simulink model "EMS"  (R2024b)
settings: configuration reference "STM32H7_Config" (kept outside this file)
undefined symbols (not defined in the file): rEMSTarget
libraries: simulink x4
settings Model: DataDictionary=Master_Dictionary.sldd  EnableAccessToBaseWorkspace=off  Creator=torni  LastModifiedBy=William
settings ConfigSetRef: SourceName=STM32H7_Config

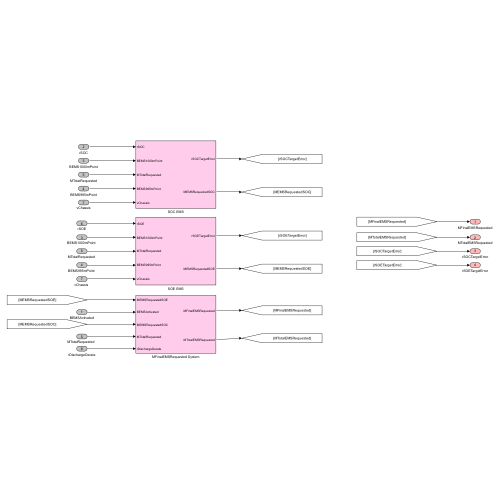
[thumbnail: Simulink's stored preview of the top-level diagram]
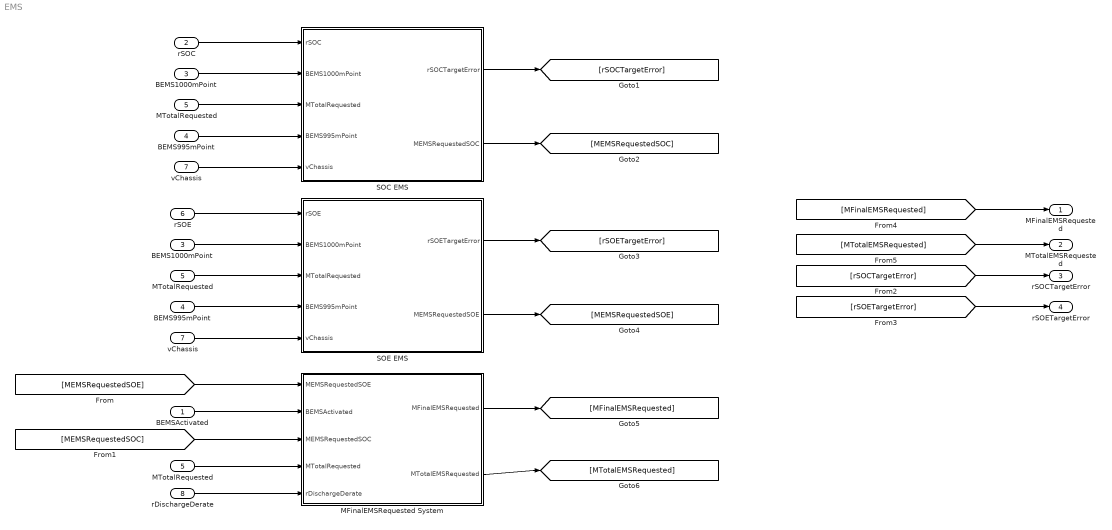
== system EMS ==
  BEMSActivated : Inport  OutDataTypeStr=boolean
  rSOC : Inport  Port=2  OutDataTypeStr=double
  BEMS1000mPoint : Inport  Port=3  OutDataTypeStr=boolean
  BEMS995mPoint : Inport  Port=4  OutDataTypeStr=boolean
  MTotalRequested : Inport  Port=5  OutDataTypeStr=double
  rSOE : Inport  Port=6  OutDataTypeStr=double
  vChassis : Inport  Port=7  OutDataTypeStr=double
  rDischargeDerate : Inport  Port=8  OutDataTypeStr=double
  "BEMS1000mPoint " : InportShadow  Port=3  OutDataTypeStr=boolean
  "BEMS995mPoint " : InportShadow  Port=4  OutDataTypeStr=boolean
  MFinalEMSRequested System : Subsystem
  "MTotalRequested " : InportShadow  Port=5  OutDataTypeStr=double
  "MTotalRequested  " : InportShadow  Port=5  OutDataTypeStr=double
  SOC EMS : Subsystem
  SOE EMS : Subsystem
  "vChassis " : InportShadow  Port=7  OutDataTypeStr=double
  MFinalEMSRequested : Outport  OutDataTypeStr=double  VectorParamsAs1DForOutWhenUnconnected=off
  MTotalEMSRequested : Outport  Port=2  OutDataTypeStr=double  VectorParamsAs1DForOutWhenUnconnected=off
  rSOCTargetError : Outport  Port=3  OutDataTypeStr=double  VectorParamsAs1DForOutWhenUnconnected=off
  rSOETargetError : Outport  Port=4  OutDataTypeStr=double  VectorParamsAs1DForOutWhenUnconnected=off
  wires:
  [rSOETargetError] -> rSOETargetError/1
  [rSOCTargetError] -> rSOCTargetError/1
  rSOC/1 -> SOC EMS/1(rSOC)
  BEMS1000mPoint/1 -> SOC EMS/2(BEMS1000mPoint)
  BEMS995mPoint/1 -> SOC EMS/4(BEMS995mPoint)
  MTotalRequested/1 -> SOC EMS/3(MTotalRequested)
  rSOE/1 -> SOE EMS/1(rSOE)
  "BEMS1000mPoint "/1 -> SOE EMS/2(BEMS1000mPoint)
  "BEMS995mPoint "/1 -> SOE EMS/4(BEMS995mPoint)
  "MTotalRequested "/1 -> SOE EMS/3(MTotalRequested)
  SOC EMS/1(rSOCTargetError) -> [rSOCTargetError]
  SOC EMS/2(MEMSRequestedSOC) -> [MEMSRequestedSOC]
  SOE EMS/1(rSOETargetError) -> [rSOETargetError]
  SOE EMS/2(MEMSRequestedSOE) -> [MEMSRequestedSOE]
  BEMSActivated/1 -> MFinalEMSRequested System/2(BEMSActivated)
  "MTotalRequested  "/1 -> MFinalEMSRequested System/4(MTotalRequested)
  [MEMSRequestedSOE] -> MFinalEMSRequested System/1(MEMSRequestedSOE)
  [MEMSRequestedSOC] -> MFinalEMSRequested System/3(MEMSRequestedSOC)
  MFinalEMSRequested System/1(MFinalEMSRequested) -> [MFinalEMSRequested]
  MFinalEMSRequested System/2(MTotalEMSRequested) -> [MTotalEMSRequested]
  [MFinalEMSRequested] -> MFinalEMSRequested/1
  [MTotalEMSRequested] -> MTotalEMSRequested/1
  vChassis/1 -> SOC EMS/5(vChassis)
  "vChassis "/1 -> SOE EMS/5(vChassis)
  rDischargeDerate/1 -> MFinalEMSRequested System/5(rDischargeDerate)

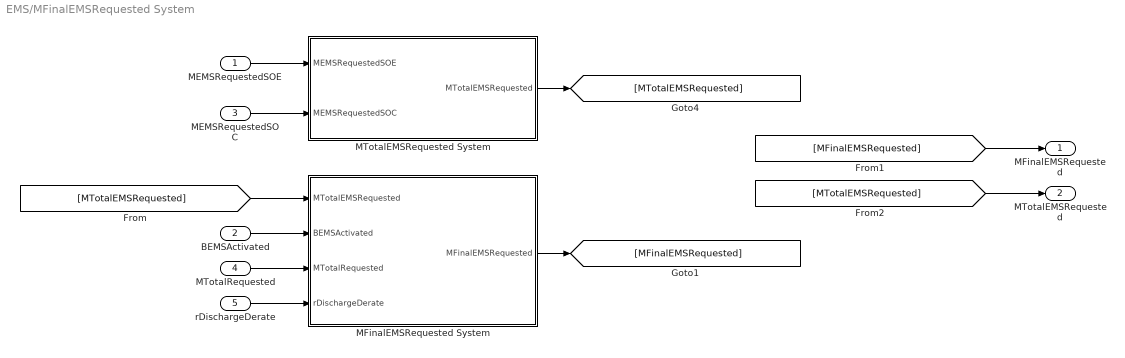
== system EMS/MFinalEMSRequested System ==
  MEMSRequestedSOE : Inport  OutDataTypeStr=double
  BEMSActivated : Inport  Port=2  OutDataTypeStr=boolean
  MEMSRequestedSOC : Inport  Port=3  OutDataTypeStr=double
  MTotalRequested : Inport  Port=4  OutDataTypeStr=double
  rDischargeDerate : Inport  Port=5  OutDataTypeStr=double
  MFinalEMSRequested System : Subsystem
  MTotalEMSRequested System : Subsystem
  MFinalEMSRequested : Outport  OutDataTypeStr=double  VectorParamsAs1DForOutWhenUnconnected=off
  MTotalEMSRequested : Outport  Port=2  OutDataTypeStr=double  VectorParamsAs1DForOutWhenUnconnected=off
  wires:
  [MTotalEMSRequested] -> MTotalEMSRequested/1
  MEMSRequestedSOE/1 -> MTotalEMSRequested System/1(MEMSRequestedSOE)
  MEMSRequestedSOC/1 -> MTotalEMSRequested System/2(MEMSRequestedSOC)
  MTotalEMSRequested System/1(MTotalEMSRequested) -> [MTotalEMSRequested]
  BEMSActivated/1 -> MFinalEMSRequested System/2(BEMSActivated)
  MTotalRequested/1 -> MFinalEMSRequested System/3(MTotalRequested)
  MFinalEMSRequested System/1(MFinalEMSRequested) -> [MFinalEMSRequested]
  [MTotalEMSRequested] -> MFinalEMSRequested System/1(MTotalEMSRequested)
  [MFinalEMSRequested] -> MFinalEMSRequested/1
  rDischargeDerate/1 -> MFinalEMSRequested System/4(rDischargeDerate)

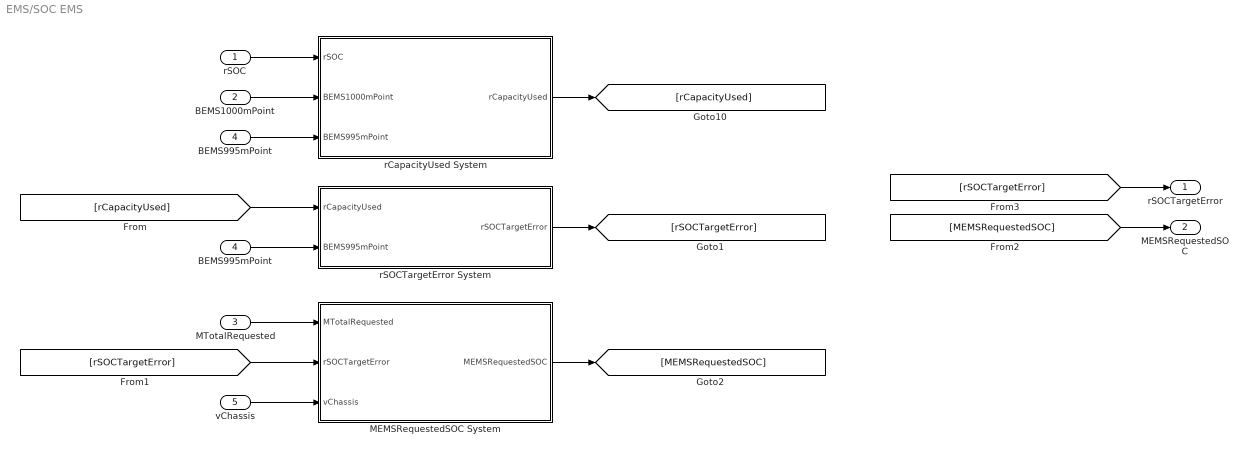
== system EMS/SOC EMS ==
  rSOC : Inport  OutDataTypeStr=double
  BEMS1000mPoint : Inport  Port=2  OutDataTypeStr=boolean
  MTotalRequested : Inport  Port=3  OutDataTypeStr=double
  BEMS995mPoint : Inport  Port=4  OutDataTypeStr=boolean
  vChassis : Inport  Port=5  OutDataTypeStr=double
  "BEMS995mPoint " : InportShadow  Port=4  OutDataTypeStr=boolean
  MEMSRequestedSOC System : Subsystem
  rCapacityUsed System : Subsystem
  rSOCTargetError System : Subsystem
  rSOCTargetError : Outport  OutDataTypeStr=double  VectorParamsAs1DForOutWhenUnconnected=off
  MEMSRequestedSOC : Outport  Port=2  OutDataTypeStr=double
  wires:
  BEMS995mPoint/1 -> rCapacityUsed System/3(BEMS995mPoint)
  MTotalRequested/1 -> MEMSRequestedSOC System/1(MTotalRequested)
  MEMSRequestedSOC System/1(MEMSRequestedSOC) -> [MEMSRequestedSOC]
  BEMS1000mPoint/1 -> rCapacityUsed System/2(BEMS1000mPoint)
  rSOC/1 -> rCapacityUsed System/1(rSOC)
  rCapacityUsed System/1(rCapacityUsed) -> [rCapacityUsed]
  [rCapacityUsed] -> rSOCTargetError System/1(rCapacityUsed)
  "BEMS995mPoint "/1 -> rSOCTargetError System/2(BEMS995mPoint)
  rSOCTargetError System/1(rSOCTargetError) -> [rSOCTargetError]
  [rSOCTargetError] -> MEMSRequestedSOC System/2(rSOCTargetError)
  [MEMSRequestedSOC] -> MEMSRequestedSOC/1
  [rSOCTargetError] -> rSOCTargetError/1
  vChassis/1 -> MEMSRequestedSOC System/3(vChassis)

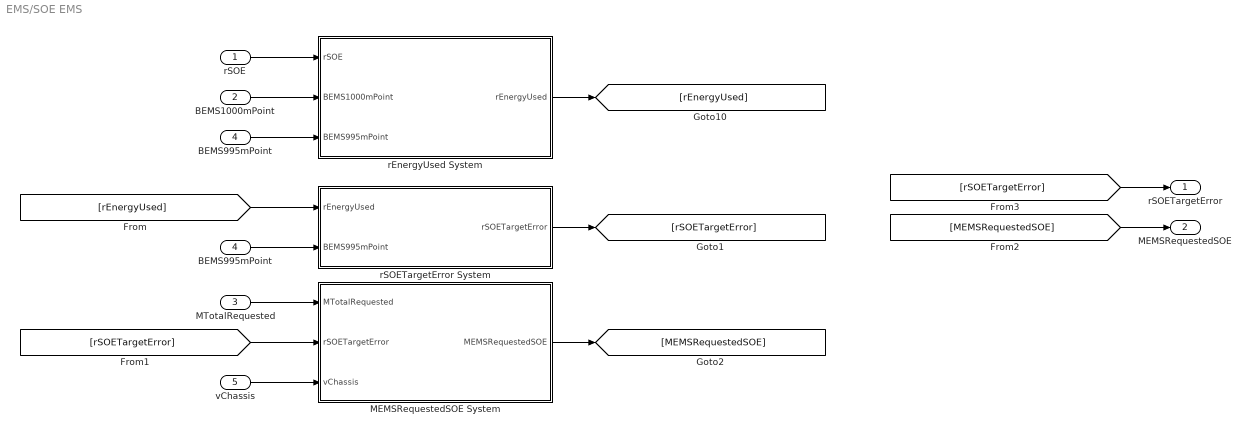
== system EMS/SOE EMS ==
  rSOE : Inport  OutDataTypeStr=double
  BEMS1000mPoint : Inport  Port=2  OutDataTypeStr=boolean
  MTotalRequested : Inport  Port=3  OutDataTypeStr=double
  BEMS995mPoint : Inport  Port=4  OutDataTypeStr=boolean
  vChassis : Inport  Port=5  OutDataTypeStr=double
  "BEMS995mPoint " : InportShadow  Port=4  OutDataTypeStr=boolean
  MEMSRequestedSOE System : Subsystem
  rEnergyUsed System : Subsystem
  rSOETargetError System : Subsystem
  rSOETargetError : Outport  OutDataTypeStr=double  VectorParamsAs1DForOutWhenUnconnected=off
  MEMSRequestedSOE : Outport  Port=2  OutDataTypeStr=double
  wires:
  [rSOETargetError] -> rSOETargetError/1
  [MEMSRequestedSOE] -> MEMSRequestedSOE/1
  [rSOETargetError] -> MEMSRequestedSOE System/2(rSOETargetError)
  rSOETargetError System/1(rSOETargetError) -> [rSOETargetError]
  "BEMS995mPoint "/1 -> rSOETargetError System/2(BEMS995mPoint)
  [rEnergyUsed] -> rSOETargetError System/1(rEnergyUsed)
  rEnergyUsed System/1(rEnergyUsed) -> [rEnergyUsed]
  rSOE/1 -> rEnergyUsed System/1(rSOE)
  BEMS1000mPoint/1 -> rEnergyUsed System/2(BEMS1000mPoint)
  MEMSRequestedSOE System/1(MEMSRequestedSOE) -> [MEMSRequestedSOE]
  MTotalRequested/1 -> MEMSRequestedSOE System/1(MTotalRequested)
  BEMS995mPoint/1 -> rEnergyUsed System/3(BEMS995mPoint)
  vChassis/1 -> MEMSRequestedSOE System/3(vChassis)

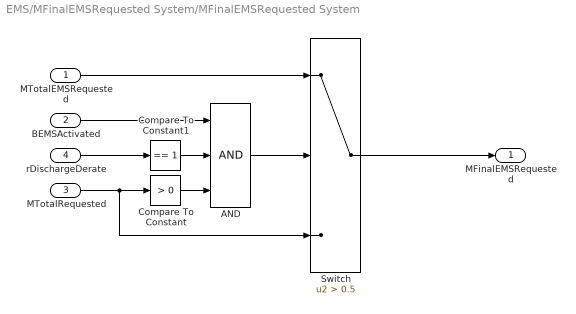
== system EMS/MFinalEMSRequested System/MFinalEMSRequested System ==
  MTotalEMSRequested : Inport  OutDataTypeStr=double
  BEMSActivated : Inport  Port=2  OutDataTypeStr=boolean
  MTotalRequested : Inport  Port=3  OutDataTypeStr=double
  rDischargeDerate : Inport  Port=4  OutDataTypeStr=double
  AND : Logic  Inputs=3  AllPortsSameDT=off  OutDataTypeStr=boolean
  Compare To Constant : simulink/Logic and Bit Operations/Compare To Constant  relop=>  const=0  OutDataTypeStr=boolean
  Compare To Constant1 : simulink/Logic and Bit Operations/Compare To Constant  relop===  const=1  OutDataTypeStr=boolean
  Switch : Switch  Criteria=u2 > Threshold  Threshold=0.5  SaturateOnIntegerOverflow=off  InputSameDT=off
  MFinalEMSRequested : Outport  OutDataTypeStr=double  VectorParamsAs1DForOutWhenUnconnected=off
  wires:
  MTotalEMSRequested/1 -> Switch/1
  MTotalRequested/1 -> Switch/3, Compare To Constant/1
  AND/1 -> Switch/2
  BEMSActivated/1 -> AND/1
  Switch/1 -> MFinalEMSRequested/1
  Compare To Constant/1 -> AND/3
  rDischargeDerate/1 -> Compare To Constant1/1
  Compare To Constant1/1 -> AND/2

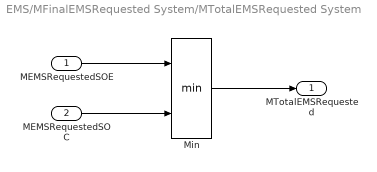
== system EMS/MFinalEMSRequested System/MTotalEMSRequested System ==
  MEMSRequestedSOE : Inport  OutDataTypeStr=double
  MEMSRequestedSOC : Inport  Port=2  OutDataTypeStr=double
  Min : MinMax  Inputs=2
  MTotalEMSRequested : Outport  OutDataTypeStr=double  VectorParamsAs1DForOutWhenUnconnected=off
  wires:
  MEMSRequestedSOE/1 -> Min/1
  MEMSRequestedSOC/1 -> Min/2
  Min/1 -> MTotalEMSRequested/1

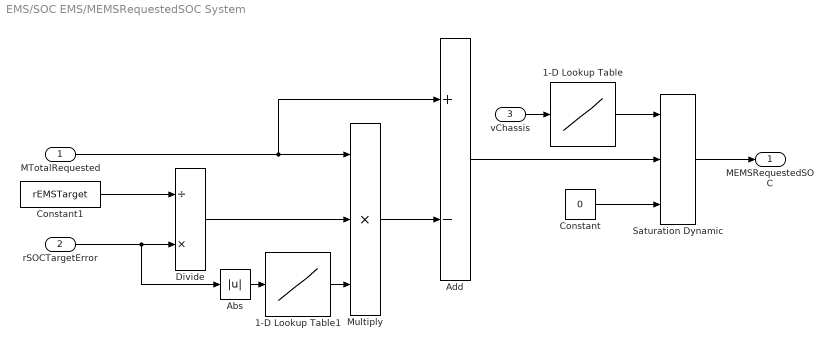
== system EMS/SOC EMS/MEMSRequestedSOC System ==
  MTotalRequested : Inport  OutDataTypeStr=double
  rSOCTargetError : Inport  Port=2  OutDataTypeStr=double
  vChassis : Inport  Port=3  OutDataTypeStr=double
  1-D Lookup Table : Lookup_n-D  NumberOfTableDimensions=1  BreakpointsForDimension1=|  Table=|  InternalRulePriority=Speed  RndMeth=Simplest
      BreakpointsForDimension1=|
      | [0.00
      | 1.37
      | 2.73
      | 4.10
      | 5.47
      | 6.84
      | 8.20
      | 9.57
      | 10.94
      | 12.30
      | 13.67
      | 15.04
      | 16.40
      | 17.77
      | 19.14
      | 20.51
      | 21.87
      | 23.24
      | 24.61
      | 25.97
      | 27.34]
      Table=|
      | [583.09
      | 583.09
      | 583.09
      | 583.09
      | 583.09
      | 583.09
      | 583.09
      | 583.09
      | 583.09
      | 583.09
      | 583.09
      | 523.483965
      | 463.877551
      | 463.877551
      | 463.877551
      | 463.877551
      | 463.877551
      | 463.877551
      | 463.877551
      | 463.877551
      | 463.877551]
  1-D Lookup Table1 : Lookup_n-D  NumberOfTableDimensions=1  BreakpointsForDimension1=[0 5]  Table=[0 3.8]  InternalRulePriority=Speed  RndMeth=Simplest
  Abs : Abs  SaturateOnIntegerOverflow=off
  Add : Sum  Inputs=+-
  Constant : Constant  Value=0
  Constant1 : Constant  Value=rEMSTarget
  Divide : Product  Inputs=/*
  Multiply : Product  Inputs=3
  Saturation Dynamic : simulink/Discontinuities/Saturation Dynamic  OutMin=[]  OutMax=[]  OutDataTypeStr=Inherit: Same as second input  OutDataType=fixdt(1, 16)  OutScaling=2^-10  DoSatur=off
  MEMSRequestedSOC : Outport  OutDataTypeStr=double
  wires:
  MTotalRequested/1 -> Add/1, Multiply/1
  Divide/1 -> Multiply/2
  Constant1/1 -> Divide/1
  rSOCTargetError/1 -> Abs/1, Divide/2
  Multiply/1 -> Add/2
  Add/1 -> Saturation Dynamic/2
  Saturation Dynamic/1 -> MEMSRequestedSOC/1
  1-D Lookup Table1/1 -> Multiply/3
  1-D Lookup Table/1 -> Saturation Dynamic/1
  vChassis/1 -> 1-D Lookup Table/1
  Constant/1 -> Saturation Dynamic/3
  Abs/1 -> 1-D Lookup Table1/1

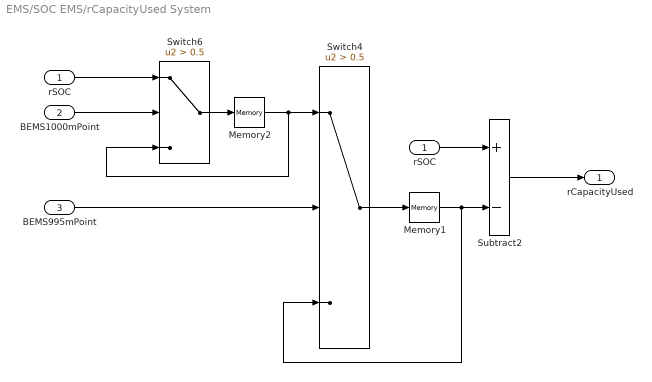
== system EMS/SOC EMS/rCapacityUsed System ==
  rSOC : Inport  OutDataTypeStr=double
  BEMS1000mPoint : Inport  Port=2  OutDataTypeStr=boolean
  BEMS995mPoint : Inport  Port=3  OutDataTypeStr=boolean
  Memory1 : Memory  InitialCondition=100  InheritSampleTime=on
  Memory2 : Memory  InitialCondition=100  InheritSampleTime=on
  Subtract2 : Sum  Inputs=+-
  Switch4 : Switch  Criteria=u2 > Threshold  Threshold=0.5  SaturateOnIntegerOverflow=off  InputSameDT=off
  Switch6 : Switch  Criteria=u2 > Threshold  Threshold=0.5  SaturateOnIntegerOverflow=off  InputSameDT=off
  "rSOC " : InportShadow  OutDataTypeStr=double
  rCapacityUsed : Outport  OutDataTypeStr=double  VectorParamsAs1DForOutWhenUnconnected=off
  wires:
  BEMS1000mPoint/1 -> Switch6/2
  Memory1/1 -> Switch4/3, Subtract2/2
  Switch4/1 -> Memory1/1
  BEMS995mPoint/1 -> Switch4/2
  rSOC/1 -> Switch6/1
  Switch6/1 -> Memory2/1
  Subtract2/1 -> rCapacityUsed/1
  Memory2/1 -> Switch6/3, Switch4/1
  "rSOC "/1 -> Subtract2/1

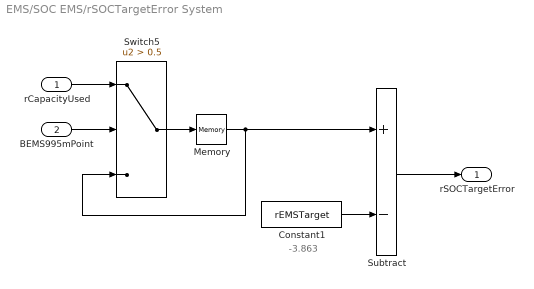
== system EMS/SOC EMS/rSOCTargetError System ==
  note: -3.863
  rCapacityUsed : Inport  OutDataTypeStr=double
  BEMS995mPoint : Inport  Port=2  OutDataTypeStr=boolean
  Constant1 : Constant  Value=rEMSTarget
  Memory : Memory  InitialCondition=-3.863  InheritSampleTime=on
  Subtract : Sum  Inputs=+-
  Switch5 : Switch  Criteria=u2 > Threshold  Threshold=0.5  SaturateOnIntegerOverflow=off  InputSameDT=off
  rSOCTargetError : Outport  OutDataTypeStr=double  VectorParamsAs1DForOutWhenUnconnected=off
  wires:
  rCapacityUsed/1 -> Switch5/1
  Switch5/1 -> Memory/1
  Constant1/1 -> Subtract/2
  BEMS995mPoint/1 -> Switch5/2
  Memory/1 -> Switch5/3, Subtract/1
  Subtract/1 -> rSOCTargetError/1

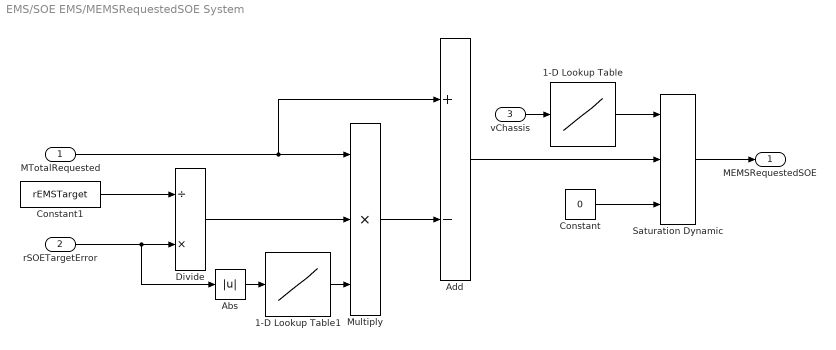
== system EMS/SOE EMS/MEMSRequestedSOE System ==
  MTotalRequested : Inport  OutDataTypeStr=double
  rSOETargetError : Inport  Port=2  OutDataTypeStr=double
  vChassis : Inport  Port=3  OutDataTypeStr=double
  1-D Lookup Table : Lookup_n-D  NumberOfTableDimensions=1  BreakpointsForDimension1=|  Table=|  InternalRulePriority=Speed  RndMeth=Simplest
      BreakpointsForDimension1=|
      | [0.00
      | 1.37
      | 2.73
      | 4.10
      | 5.47
      | 6.84
      | 8.20
      | 9.57
      | 10.94
      | 12.30
      | 13.67
      | 15.04
      | 16.40
      | 17.77
      | 19.14
      | 20.51
      | 21.87
      | 23.24
      | 24.61
      | 25.97
      | 27.34]
      Table=|
      | [583.09
      | 583.09
      | 583.09
      | 583.09
      | 583.09
      | 583.09
      | 583.09
      | 583.09
      | 509.86
      | 509.86
      | 509.86
      | 509.8639456
      | 509.8639456
      | 509.8639456
      | 509.8639456
      | 509.8639456
      | 509.8639456
      | 509.8639456
      | 509.8639456
      | 509.8639456
      | 509.8639456]
  1-D Lookup Table1 : Lookup_n-D  NumberOfTableDimensions=1  BreakpointsForDimension1=[0 5]  Table=[0 3.8]  InternalRulePriority=Speed  RndMeth=Simplest
  Abs : Abs  SaturateOnIntegerOverflow=off
  Add : Sum  Inputs=+-
  Constant : Constant  Value=0
  Constant1 : Constant  Value=rEMSTarget
  Divide : Product  Inputs=/*
  Multiply : Product  Inputs=3
  Saturation Dynamic : simulink/Discontinuities/Saturation Dynamic  OutMin=[]  OutMax=[]  OutDataTypeStr=Inherit: Same as second input  OutDataType=fixdt(1, 16)  OutScaling=2^-10  DoSatur=off
  MEMSRequestedSOE : Outport  OutDataTypeStr=double
  wires:
  MTotalRequested/1 -> Add/1, Multiply/1
  Divide/1 -> Multiply/2
  Constant1/1 -> Divide/1
  rSOETargetError/1 -> Abs/1, Divide/2
  Multiply/1 -> Add/2
  Add/1 -> Saturation Dynamic/2
  Saturation Dynamic/1 -> MEMSRequestedSOE/1
  1-D Lookup Table1/1 -> Multiply/3
  1-D Lookup Table/1 -> Saturation Dynamic/1
  vChassis/1 -> 1-D Lookup Table/1
  Constant/1 -> Saturation Dynamic/3
  Abs/1 -> 1-D Lookup Table1/1

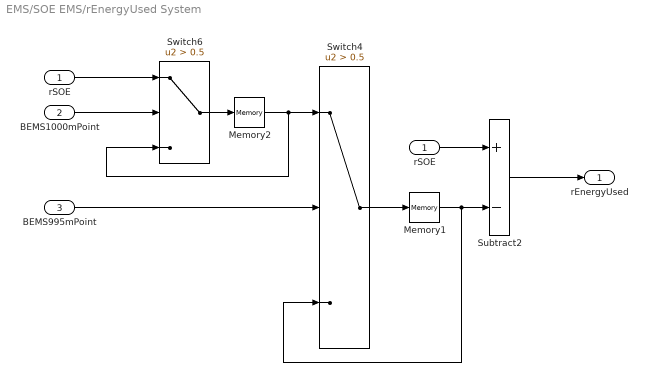
== system EMS/SOE EMS/rEnergyUsed System ==
  rSOE : Inport  OutDataTypeStr=double
  BEMS1000mPoint : Inport  Port=2  OutDataTypeStr=boolean
  BEMS995mPoint : Inport  Port=3  OutDataTypeStr=boolean
  Memory1 : Memory  InitialCondition=100  InheritSampleTime=on
  Memory2 : Memory  InitialCondition=100  InheritSampleTime=on
  Subtract2 : Sum  Inputs=+-
  Switch4 : Switch  Criteria=u2 > Threshold  Threshold=0.5  SaturateOnIntegerOverflow=off  InputSameDT=off
  Switch6 : Switch  Criteria=u2 > Threshold  Threshold=0.5  SaturateOnIntegerOverflow=off  InputSameDT=off
  "rSOE " : InportShadow  OutDataTypeStr=double
  rEnergyUsed : Outport  OutDataTypeStr=double  VectorParamsAs1DForOutWhenUnconnected=off
  wires:
  "rSOE "/1 -> Subtract2/1
  Memory2/1 -> Switch4/1, Switch6/3
  Subtract2/1 -> rEnergyUsed/1
  Switch6/1 -> Memory2/1
  rSOE/1 -> Switch6/1
  BEMS995mPoint/1 -> Switch4/2
  Switch4/1 -> Memory1/1
  Memory1/1 -> Subtract2/2, Switch4/3
  BEMS1000mPoint/1 -> Switch6/2

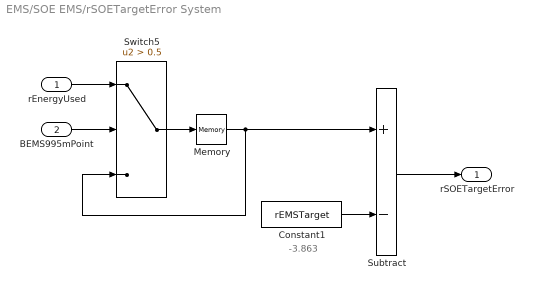
== system EMS/SOE EMS/rSOETargetError System ==
  note: -3.863
  rEnergyUsed : Inport  OutDataTypeStr=double
  BEMS995mPoint : Inport  Port=2  OutDataTypeStr=boolean
  Constant1 : Constant  Value=rEMSTarget
  Memory : Memory  InitialCondition=-3.863  InheritSampleTime=on
  Subtract : Sum  Inputs=+-
  Switch5 : Switch  Criteria=u2 > Threshold  Threshold=0.5  SaturateOnIntegerOverflow=off  InputSameDT=off
  rSOETargetError : Outport  OutDataTypeStr=double  VectorParamsAs1DForOutWhenUnconnected=off
  wires:
  Subtract/1 -> rSOETargetError/1
  Memory/1 -> Subtract/1, Switch5/3
  BEMS995mPoint/1 -> Switch5/2
  Constant1/1 -> Subtract/2
  Switch5/1 -> Memory/1
  rEnergyUsed/1 -> Switch5/1
